simulink library "pwrsys"  (R2018a)
settings: Solver=VariableStepAuto  StartTime=0.0  StopTime=10.0  RelTol=1e-3
values from neighbouring files (symbols this model uses):
  Ts = Ts_c    (= 1e-07)    [PlantStateEquations_abc_Script.m]
undefined symbols (not defined in the file or in its folder): D1, Delta, DiscIntNeverNeededParam, ESS, f_LPF_noise, fn, fsw, grid, gt1, Iap, Kp, PCC, Refmax, Refmin, sim, SIMU, Sn, tctrl, Ti, Ts_control, Ts_PWM, Uabp, Uanp, WT, X, zeta
libraries: $bdroot x71, powerlib x59, powerlib_meascontrol x49, peTransforms x20, PhD_Library x1, sps_avr x1
(part 4 of 4)

== system pwrsys/Voltage and Current Controllers/DualRegulator ==
  idqref : Inport
  vabc : Inport  Port=2
  iabc : Inport  Port=3
  wt : Inport  Port=4
  w_pu : Inport  Port=5
  Udc : Inport  Port=6
  1=enable_acb : Inport  Port=7
  1=no,2=Notch,3=DSC : Inport  Port=8
  pre_mult_PI_errors : Inport  Port=9
  force_int : Inport  Port=10
  force_val : Inport  Port=11
  Bus Creator : BusCreator  Inputs=4
  Constant1 : Constant  Value=0
  Constant10 : Constant
  Constant14 : Constant
  Constant18 : Constant  Value=[0 0]
  Constant6 : Constant
  Constant8 : Constant  Value=0
  Idq_Dec_Signs_Fdbk_Ref : $bdroot/Voltage and Current Controllers/Idq_Dec_Signs_Fdbk_Ref  Ts=Ts  fn=fgrid  Kp=PI_Kp  Ti=PI_Ti  L=PI_X  PI_max=PI_max  PI_min=PI_min  TrafoPhaseComp=0
  Idq_Dec_Signs_Fdbk_Ref_acb : $bdroot/Voltage and Current Controllers/Idq_Dec_Signs_Fdbk_Ref  Ts=Ts  fn=fgrid  Kp=PI_Kp  Ti=PI_Ti  L=PI_X  PI_max=PI_max  PI_min=PI_min  TrafoPhaseComp=0
  PWM_abc_negwt_acb : $bdroot/PWM/PWM_abc_negwt_acb  fsw=PWM_fsw  Ts=PWM_Ts  Uabp=PWM_Uabp  PWM_Ini_Phase=PWM_Ini
  Selector1 : Selector  InputPortWidth=3  IndexOptions=Index vector (dialog)  Indices=[1 3 2]  OutputSizes=1
  Selector7 : Selector  InputPortWidth=3  IndexOptions=Index vector (dialog)  Indices=[1 3 2]  OutputSizes=1
  Terminator{1..4,24} (5 alike) : Terminator
  abc_dq_bypassnotch1 : $bdroot/Transformations/abc_dq_bypassnotch  Ts=Ts  fn=2*fgrid  fcutoutv=fcutoutLPF  fcutouti=fcutoutLPF  zeta=zetanotch
  abc_dq_bypassnotch2 : $bdroot/Transformations/abc_dq_bypassnotch  Ts=Ts  fn=2*fgrid  fcutoutv=fcutoutLPF  fcutouti=fcutoutLPF  zeta=zetanotch
  idqref_gen_for_cnst_p : $bdroot/Voltage and Current Controllers/idqref_gen_for_cnst_p  Ts_control=Ts
  PWMpulses : Outport
  Uabcref : Outport  Port=2
  mvidq : Outport  Port=3
  mpi+ : Outport  Port=4
  mpi- : Outport  Port=5
  wires:
  Udc/1 -> PWM_abc_negwt_acb/7
  abc_dq_bypassnotch1/1 -> idqref_gen_for_cnst_p/2, Bus Creator/3, Idq_Dec_Signs_Fdbk_Ref_acb/2  "vdq-"
  [w_pu] -> Idq_Dec_Signs_Fdbk_Ref/4
  PWM_abc_negwt_acb/3 -> Terminator24/1
  Constant14/1 -> Idq_Dec_Signs_Fdbk_Ref_acb/5
  abc_dq_bypassnotch2/1 -> idqref_gen_for_cnst_p/1, Bus Creator/1, Idq_Dec_Signs_Fdbk_Ref/2  "vdq+"
  abc_dq_bypassnotch1/2 -> Bus Creator/4, Idq_Dec_Signs_Fdbk_Ref_acb/3  "idq-"
  Constant10/1 -> PWM_abc_negwt_acb/2
  Constant8/1 -> PWM_abc_negwt_acb/4
  abc_dq_bypassnotch2/2 -> Bus Creator/2, Idq_Dec_Signs_Fdbk_Ref/3  "idq+"
  1=enable_acb/1 -> PWM_abc_negwt_acb/6
  Idq_Dec_Signs_Fdbk_Ref/1 -> PWM_abc_negwt_acb/1
  PWM_abc_negwt_acb/1 -> PWMpulses/1
  PWM_abc_negwt_acb/2 -> Uabcref/1  "Uabcref"
  Constant6/1 -> Idq_Dec_Signs_Fdbk_Ref/5
  Constant1/1 -> Idq_Dec_Signs_Fdbk_Ref_acb/6, Idq_Dec_Signs_Fdbk_Ref/6
  vabc/1 -> abc_dq_bypassnotch2/1, Selector7/1
  iabc/1 -> abc_dq_bypassnotch2/2, Selector1/1
  Idq_Dec_Signs_Fdbk_Ref_acb/1 -> PWM_abc_negwt_acb/5
  wt/1 -> abc_dq_bypassnotch2/3, abc_dq_bypassnotch1/3, [theta]
  Selector7/1 -> abc_dq_bypassnotch1/1
  Selector1/1 -> abc_dq_bypassnotch1/2
  Constant18/1 -> PWM_abc_negwt_acb/3
  idqref/1 -> idqref_gen_for_cnst_p/3, Idq_Dec_Signs_Fdbk_Ref/1
  idqref_gen_for_cnst_p/1 -> Idq_Dec_Signs_Fdbk_Ref_acb/1
  [theta] -> PWM_abc_negwt_acb/8
  1=no,2=Notch,3=DSC/1 -> abc_dq_bypassnotch2/5, abc_dq_bypassnotch1/5
  Bus Creator/1 -> mvidq/1
  w_pu/1 -> abc_dq_bypassnotch2/4, abc_dq_bypassnotch1/4, [w_pu]
  [w_pu] -> Idq_Dec_Signs_Fdbk_Ref_acb/4
  pre_mult_PI_errors/1 -> Idq_Dec_Signs_Fdbk_Ref_acb/7, Idq_Dec_Signs_Fdbk_Ref/7
  force_int/1 -> Idq_Dec_Signs_Fdbk_Ref_acb/8, Idq_Dec_Signs_Fdbk_Ref/8
  force_val/1 -> Idq_Dec_Signs_Fdbk_Ref_acb/10, Idq_Dec_Signs_Fdbk_Ref_acb/9, Idq_Dec_Signs_Fdbk_Ref/10, Idq_Dec_Signs_Fdbk_Ref/9
  Idq_Dec_Signs_Fdbk_Ref/4 -> mpi+/1
  Idq_Dec_Signs_Fdbk_Ref_acb/4 -> mpi-/1
  Idq_Dec_Signs_Fdbk_Ref/2 -> Terminator1/1
  Idq_Dec_Signs_Fdbk_Ref/3 -> Terminator2/1
  Idq_Dec_Signs_Fdbk_Ref_acb/2 -> Terminator3/1
  Idq_Dec_Signs_Fdbk_Ref_acb/3 -> Terminator4/1

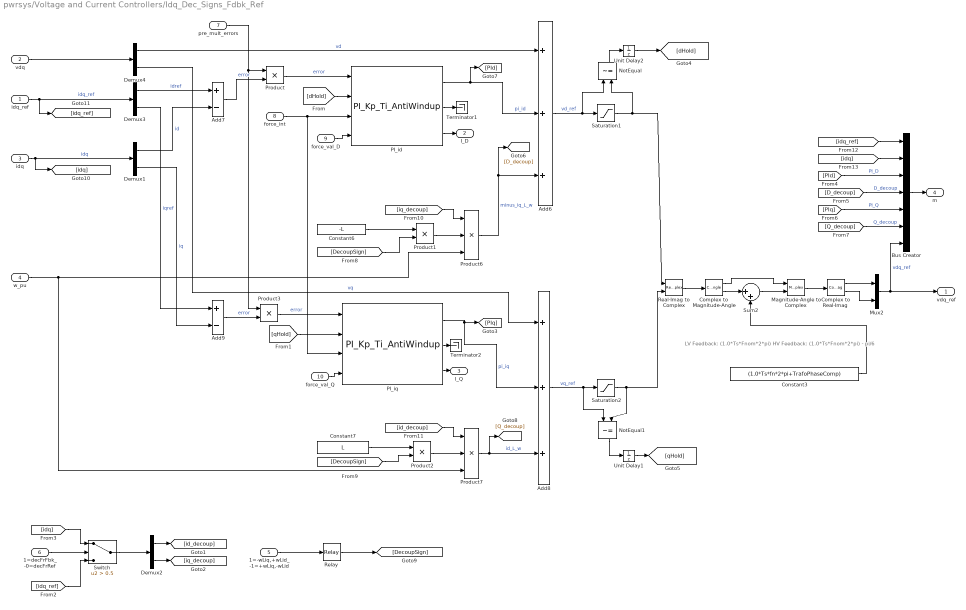
== system pwrsys/Voltage and Current Controllers/Idq_Dec_Signs_Fdbk_Ref ==
  note: LV Feedback: (1.0*Ts*Fnom*2*pi)
      | HV Feedback: (1.0*Ts*Fnom*2*pi) - pi/6
  idq_ref : Inport
  vdq : Inport  Port=2
  idq : Inport  Port=3
  w_pu : Inport  Port=4
  1=-wLiq,+wLid_-1=+wLiq,-wLid : Inport  Port=5
  1=decFrFbk_-0=decFrRef : Inport  Port=6
  pre_mult_errors : Inport  Port=7
  force_int : Inport  Port=8
  force_val_D : Inport  Port=9
  force_val_Q : Inport  Port=10
  Add6 : Sum  Inputs=+++
  Add7 : Sum  Inputs=+-
  Add8 : Sum  Inputs=+++
  Add9 : Sum  Inputs=+-
  Bus Creator : BusCreator  Inputs=7
  Complex to Magnitude-Angle : ComplexToMagnitudeAngle
  Complex to Real-Imag : ComplexToRealImag
  Constant3 : Constant  Value=(1.0*Ts*fn*2*pi+TrafoPhaseComp)  SampleTime=Ts
  Constant6 : Constant  Value=-L  SampleTime=Ts
  Constant7 : Constant  Value=L  SampleTime=Ts
  Demux{1..4} (4 alike) : Demux  Outputs=2
  Magnitude-Angle to Complex : MagnitudeAngleToComplex
  Mux2 : Mux  Inputs=2
  NotEqual : RelationalOperator  Operator=~=  OutDataTypeStr=boolean  RndMeth=Simplest
  NotEqual1 : RelationalOperator  Operator=~=  OutDataTypeStr=boolean  RndMeth=Simplest
  PI_id : $bdroot/Basic Blocks/PI_Kp_Ti_AntiWindup  Ts=Ts  Kp=Kp  Ti=Ti  PI_max=PI_max  PI_min=PI_min
  PI_iq : $bdroot/Basic Blocks/PI_Kp_Ti_AntiWindup  Ts=Ts  Kp=Kp  Ti=Ti  PI_max=PI_max  PI_min=PI_min
  Product : Product
  Product1 : Product  RndMeth=Zero
  Product2 : Product  RndMeth=Zero
  Product3 : Product
  Product6 : Product  Inputs=3  RndMeth=Zero
  Product7 : Product  Inputs=3  RndMeth=Zero
  Real-Imag to Complex : RealImagToComplex
  Relay : Relay  OnSwitchValue=0  OffSwitchValue=-0.1  OffOutputValue=-1
  Saturation1 : Saturate  UpperLimit=PI_max  LowerLimit=PI_min
  Saturation2 : Saturate  UpperLimit=PI_max  LowerLimit=PI_min
  Sum2 : Sum  Inputs=|++
  Switch : Switch  Criteria=u2 > Threshold  Threshold=0.5
  Terminator1 : Terminator
  Terminator2 : Terminator
  Unit Delay1 : UnitDelay  SampleTime=Ts
  Unit Delay2 : UnitDelay  SampleTime=Ts
  vdq_ref : Outport
  I_D : Outport  Port=2
  I_Q : Outport  Port=3
  m : Outport  Port=4
  wires:
  PI_iq/1 -> Add8/2, [PIq]  "pi_iq"
  PI_iq/2 -> Terminator2/1
  PI_id/2 -> Terminator1/1
  w_pu/1 -> Product7/3, Product6/3
  Product3/1 -> PI_iq/1  "error"
  PI_id/1 -> Add6/2, [PId]  "pi_id"
  Constant6/1 -> Product1/1
  Constant7/1 -> Product2/1
  Demux1/1 -> Add7/2  "id"
  Product7/1 -> [Q_decoup], Add8/3  "id_L_w"
  Demux4/1 -> Add6/1  "vd"
  Product/1 -> PI_id/1  "error"
  Demux1/2 -> Add9/2  "iq"
  Product6/1 -> [D_decoup], Add6/3  "minus_iq_L_w"
  PI_iq/3 -> I_Q/1
  PI_id/3 -> I_D/1
  Demux4/2 -> Add8/1  "vq"
  Mux2/1 -> Bus Creator/7, vdq_ref/1  "vdq_ref"
  idq/1 -> [idq], Demux1/1  "idq"
  vdq/1 -> Demux4/1
  Add8/1 -> NotEqual1/1, Saturation2/1  "vq_ref"
  Add6/1 -> NotEqual/1, Saturation1/1  "vd_ref"
  idq_ref/1 -> [idq_ref], Demux3/1  "idq_ref"
  Demux3/1 -> Add7/1  "idref"
  Demux3/2 -> Add9/1  "iqref"
  Magnitude-Angle to Complex/1 -> Complex to Real-Imag/1
  Real-Imag to Complex/1 -> Complex to Magnitude-Angle/1
  Complex to Magnitude-Angle/1 -> Magnitude-Angle to Complex/1
  Complex to Magnitude-Angle/2 -> Sum2/1
  Sum2/1 -> Magnitude-Angle to Complex/2
  Constant3/1 -> Sum2/2
  Complex to Real-Imag/1 -> Mux2/1
  Complex to Real-Imag/2 -> Mux2/2
  [PId] -> Bus Creator/3  "PI_D"
  [D_decoup] -> Bus Creator/4  "D_decoup"
  [PIq] -> Bus Creator/5  "PI_Q"
  Bus Creator/1 -> m/1
  [Q_decoup] -> Bus Creator/6  "Q_decoup"
  Saturation1/1 -> NotEqual/2, Real-Imag to Complex/1
  NotEqual/1 -> Unit Delay2/1
  Saturation2/1 -> NotEqual1/2, Real-Imag to Complex/2
  NotEqual1/1 -> Unit Delay1/1
  Unit Delay2/1 -> [dHold]
  Unit Delay1/1 -> [qHold]
  [dHold] -> PI_id/2
  [qHold] -> PI_iq/2
  Relay/1 -> [DecoupSign]
  1=-wLiq,+wLid_-1=+wLiq,-wLid/1 -> Relay/1
  [DecoupSign] -> Product1/2
  Product1/1 -> Product6/2
  Product2/1 -> Product7/2
  [DecoupSign] -> Product2/2
  [idq_ref] -> Switch/3
  Demux2/2 -> [iq_decoup]
  1=decFrFbk_-0=decFrRef/1 -> Switch/2
  Demux2/1 -> [id_decoup]
  Switch/1 -> Demux2/1
  [idq] -> Switch/1
  [iq_decoup] -> Product6/1
  [id_decoup] -> Product7/1
  [idq_ref] -> Bus Creator/1
  [idq] -> Bus Creator/2
  force_int/1 -> PI_iq/3, PI_id/3
  force_val_D/1 -> PI_id/4
  force_val_Q/1 -> PI_iq/4
  Add9/1 -> Product3/2  "error"
  Add7/1 -> Product/2  "error"
  pre_mult_errors/1 -> Product3/1, Product/1

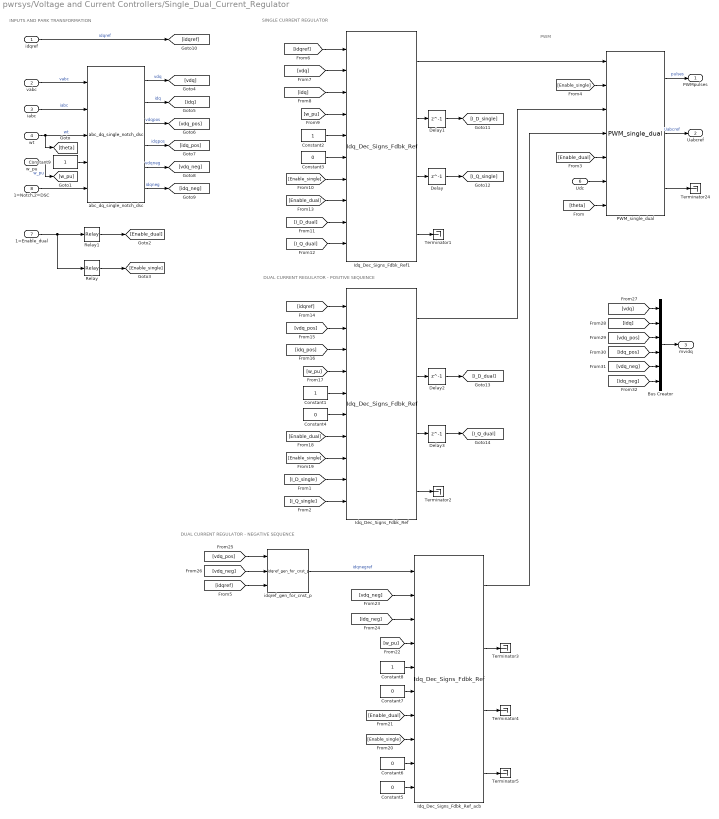
== system pwrsys/Voltage and Current Controllers/Single_Dual_Current_Regulator ==
  note: PWM
  note: DUAL CURRENT REGULATOR - NEGATIVE SEQUENCE
  note: DUAL CURRENT REGULATOR - POSITIVE SEQUENCE
  note: SINGLE CURRENT REGULATOR
  note: INPUTS AND PARK TRANSFORMATION
  idqref : Inport
  vabc : Inport  Port=2
  iabc : Inport  Port=3
  wt : Inport  Port=4
  w_pu : Inport  Port=5
  Udc : Inport  Port=6
  1=Enable_dual : Inport  Port=7
  1=Notch,2=DSC : Inport  Port=8
  Bus Creator : BusCreator  Inputs=6
  Constant{1..2,8..9} (4 alike) : Constant
  Constant{3..7} (5 alike) : Constant  Value=0
  Delay{,1..3} (4 alike) : Delay  DelayLength=1  InitialCondition=0  SampleTime=Ts
  Idq_Dec_Signs_Fdbk_Ref : $bdroot/Voltage and Current Controllers/Idq_Dec_Signs_Fdbk_Ref  Ts=Ts  fn=fgrid  Kp=PI_Kp  Ti=PI_Ti  L=PI_X  PI_max=PI_max  PI_min=PI_min  TrafoPhaseComp=0
  Idq_Dec_Signs_Fdbk_Ref1 : $bdroot/Voltage and Current Controllers/Idq_Dec_Signs_Fdbk_Ref  Ts=Ts  fn=fgrid  Kp=PI_Kp  Ti=PI_Ti  L=PI_X  PI_max=PI_max  PI_min=PI_min  TrafoPhaseComp=0
  Idq_Dec_Signs_Fdbk_Ref_acb : $bdroot/Voltage and Current Controllers/Idq_Dec_Signs_Fdbk_Ref  Ts=Ts  fn=fgrid  Kp=PI_Kp  Ti=PI_Ti  L=PI_X  PI_max=PI_max  PI_min=PI_min  TrafoPhaseComp=0
  PWM_single_dual : $bdroot/PWM/PWM_single_dual  fsw=PWM_fsw  Ts=PWM_Ts  Uabp=PWM_Uabp  PWM_Ini_Phase=PWM_Ini
  Relay : Relay  OnSwitchValue=0.6  OffSwitchValue=0.4  OnOutputValue=0  OffOutputValue=1
  Relay1 : Relay  OnSwitchValue=0.6  OffSwitchValue=0.4
  Terminator{1..5,24} (6 alike) : Terminator
  abc_dq_single_notch_dsc : $bdroot/Transformations/abc_dq_single_notch_dsc  Ts=Ts  fn=2*fgrid  zeta=zetanotch
  idqref_gen_for_cnst_p : $bdroot/Voltage and Current Controllers/idqref_gen_for_cnst_p  Ts_control=Ts
  PWMpulses : Outport
  Uabcref : Outport  Port=2
  mvidq : Outport  Port=3
  wires:
  Udc/1 -> PWM_single_dual/6
  PWM_single_dual/3 -> Terminator24/1
  PWM_single_dual/2 -> Uabcref/1  "Uabcref"
  [idqref] -> idqref_gen_for_cnst_p/3
  [theta] -> PWM_single_dual/7
  PWM_single_dual/1 -> PWMpulses/1  "pulses"
  1=Enable_dual/1 -> Relay1/1, Relay/1
  [Enable_dual] -> PWM_single_dual/5
  Relay/1 -> [Enable_single]
  [Enable_single] -> PWM_single_dual/2
  vabc/1 -> abc_dq_single_notch_dsc/1  "vabc"
  iabc/1 -> abc_dq_single_notch_dsc/2  "iabc"
  wt/1 -> [theta], abc_dq_single_notch_dsc/3  "wt"
  w_pu/1 -> [w_pu]  "w_pu"
  abc_dq_single_notch_dsc/1 -> [vdq]  "vdq"
  abc_dq_single_notch_dsc/2 -> [idq]  "idq"
  abc_dq_single_notch_dsc/3 -> [vdq_pos]  "vdqpos"
  abc_dq_single_notch_dsc/4 -> [idq_pos]  "idqpos"
  abc_dq_single_notch_dsc/5 -> [vdq_neg]  "vdqneg"
  abc_dq_single_notch_dsc/6 -> [idq_neg]  "idqneg"
  idqref/1 -> [idqref]  "idqref"
  [idqref] -> Idq_Dec_Signs_Fdbk_Ref1/1
  [vdq] -> Idq_Dec_Signs_Fdbk_Ref1/2
  [idq] -> Idq_Dec_Signs_Fdbk_Ref1/3
  [w_pu] -> Idq_Dec_Signs_Fdbk_Ref1/4
  Constant2/1 -> Idq_Dec_Signs_Fdbk_Ref1/5
  Constant3/1 -> Idq_Dec_Signs_Fdbk_Ref1/6
  Relay1/1 -> [Enable_dual]
  1=Notch,2=DSC/1 -> abc_dq_single_notch_dsc/5
  [Enable_single] -> Idq_Dec_Signs_Fdbk_Ref1/7
  Idq_Dec_Signs_Fdbk_Ref1/3 -> Delay/1
  Idq_Dec_Signs_Fdbk_Ref1/2 -> Delay1/1
  Idq_Dec_Signs_Fdbk_Ref/2 -> Delay2/1
  Idq_Dec_Signs_Fdbk_Ref/3 -> Delay3/1
  Delay1/1 -> [I_D_single]
  Delay/1 -> [I_Q_single]
  Delay2/1 -> [I_D_dual]
  Delay3/1 -> [I_Q_dual]
  [I_D_single] -> Idq_Dec_Signs_Fdbk_Ref/9
  [I_Q_single] -> Idq_Dec_Signs_Fdbk_Ref/10
  [I_D_dual] -> Idq_Dec_Signs_Fdbk_Ref1/9
  [I_Q_dual] -> Idq_Dec_Signs_Fdbk_Ref1/10
  [Enable_dual] -> Idq_Dec_Signs_Fdbk_Ref1/8
  [idqref] -> Idq_Dec_Signs_Fdbk_Ref/1
  [vdq_pos] -> Idq_Dec_Signs_Fdbk_Ref/2
  [idq_pos] -> Idq_Dec_Signs_Fdbk_Ref/3
  [w_pu] -> Idq_Dec_Signs_Fdbk_Ref/4
  Constant1/1 -> Idq_Dec_Signs_Fdbk_Ref/5
  Constant4/1 -> Idq_Dec_Signs_Fdbk_Ref/6
  [Enable_dual] -> Idq_Dec_Signs_Fdbk_Ref/7
  [Enable_single] -> Idq_Dec_Signs_Fdbk_Ref/8
  Idq_Dec_Signs_Fdbk_Ref1/4 -> Terminator1/1
  Idq_Dec_Signs_Fdbk_Ref/4 -> Terminator2/1
  Idq_Dec_Signs_Fdbk_Ref_acb/2 -> Terminator3/1
  Idq_Dec_Signs_Fdbk_Ref_acb/3 -> Terminator4/1
  Idq_Dec_Signs_Fdbk_Ref_acb/4 -> Terminator5/1
  Constant5/1 -> Idq_Dec_Signs_Fdbk_Ref_acb/10
  Constant6/1 -> Idq_Dec_Signs_Fdbk_Ref_acb/9
  [Enable_single] -> Idq_Dec_Signs_Fdbk_Ref_acb/8
  [Enable_dual] -> Idq_Dec_Signs_Fdbk_Ref_acb/7
  Constant7/1 -> Idq_Dec_Signs_Fdbk_Ref_acb/6
  Constant8/1 -> Idq_Dec_Signs_Fdbk_Ref_acb/5
  [w_pu] -> Idq_Dec_Signs_Fdbk_Ref_acb/4
  [vdq_neg] -> Idq_Dec_Signs_Fdbk_Ref_acb/2
  [idq_neg] -> Idq_Dec_Signs_Fdbk_Ref_acb/3
  [vdq_pos] -> idqref_gen_for_cnst_p/1
  [vdq_neg] -> idqref_gen_for_cnst_p/2
  idqref_gen_for_cnst_p/1 -> Idq_Dec_Signs_Fdbk_Ref_acb/1  "idqnegref"
  Idq_Dec_Signs_Fdbk_Ref1/1 -> PWM_single_dual/1
  Idq_Dec_Signs_Fdbk_Ref/1 -> PWM_single_dual/3
  Idq_Dec_Signs_Fdbk_Ref_acb/1 -> PWM_single_dual/4
  Bus Creator/1 -> mvidq/1
  [vdq] -> Bus Creator/1
  [idq] -> Bus Creator/2
  [vdq_pos] -> Bus Creator/3
  [idq_pos] -> Bus Creator/4
  [vdq_neg] -> Bus Creator/5
  [idq_neg] -> Bus Creator/6
  Constant9/1 -> abc_dq_single_notch_dsc/4

== system pwrsys/Voltage and Current Controllers/Uac_Controller ==
  vac_setpoint : Inport
  vac : Inport  Port=2
  Ihold : Inport  Port=3
  DisableP : Inport  Port=4
  pre_mult_error : Inport  Port=5
  force_int : Inport  Port=6
  force_val : Inport  Port=7
  PI_Kg_Kp_Ti_AntiWindup : $bdroot/Basic Blocks/PI_Kg_Kp_Ti_AntiWindup  Ts=Ts  Kg=Kg  Kp=Kp  Ti=Ti  PI_max=PI_max  PI_min=PI_min
  Product : Product
  Rate Transition1 : RateTransition  InitialCondition=1  OutPortSampleTime=Ts
  Rate Transition2 : RateTransition  InitialCondition=1  OutPortSampleTime=Ts
  Rate Transition3 : RateTransition  OutPortSampleTime=Ts
  Subtract : Sum  Inputs=+-
  Terminator2 : Terminator
  Terminator3 : Terminator
  iqref : Outport
  wires:
  PI_Kg_Kp_Ti_AntiWindup/2 -> Terminator2/1
  vac/1 -> Rate Transition1/1  "vac"
  PI_Kg_Kp_Ti_AntiWindup/3 -> Terminator3/1
  Subtract/1 -> Product/2
  Rate Transition1/1 -> Subtract/1
  Rate Transition2/1 -> Subtract/2
  PI_Kg_Kp_Ti_AntiWindup/1 -> iqref/1  "Idref"
  Ihold/1 -> PI_Kg_Kp_Ti_AntiWindup/3
  vac_setpoint/1 -> Rate Transition2/1
  DisableP/1 -> PI_Kg_Kp_Ti_AntiWindup/2
  force_val/1 -> PI_Kg_Kp_Ti_AntiWindup/5
  force_int/1 -> PI_Kg_Kp_Ti_AntiWindup/4
  pre_mult_error/1 -> Rate Transition3/1
  Rate Transition3/1 -> Product/1
  Product/1 -> PI_Kg_Kp_Ti_AntiWindup/1

== system pwrsys/Voltage and Current Controllers/Udc_Controller ==
  vdc : Inport
  Ihold : Inport  Port=2
  pre_mult_error : Inport  Port=3
  force_int : Inport  Port=4
  force_val : Inport  Port=5
  Constant1 : Constant
  PI_Kp_Ti_AntiWindup : $bdroot/Basic Blocks/PI_Kp_Ti_AntiWindup  Ts=Ts  Kp=Kp  Ti=Ti  PI_max=PI_max  PI_min=PI_min
  Product : Product
  Rate Transition1 : RateTransition  InitialCondition=1  OutPortSampleTime=Ts
  Rate Transition3 : RateTransition  OutPortSampleTime=Ts
  Subtract : Sum  Inputs=+-
  Terminator2 : Terminator
  Terminator3 : Terminator
  idref : Outport
  wires:
  PI_Kp_Ti_AntiWindup/2 -> Terminator2/1
  vdc/1 -> Rate Transition1/1  "vdc"
  PI_Kp_Ti_AntiWindup/3 -> Terminator3/1
  Subtract/1 -> Product/2
  Rate Transition1/1 -> Subtract/1
  Constant1/1 -> Subtract/2
  PI_Kp_Ti_AntiWindup/1 -> idref/1  "Idref"
  Ihold/1 -> PI_Kp_Ti_AntiWindup/2
  Rate Transition3/1 -> Product/1
  pre_mult_error/1 -> Rate Transition3/1
  Product/1 -> PI_Kp_Ti_AntiWindup/1
  force_int/1 -> PI_Kp_Ti_AntiWindup/3
  force_val/1 -> PI_Kp_Ti_AntiWindup/4

== system pwrsys/Voltage and Current Controllers/idqref_gen_for_cnst_p ==
  vdq+ : Inport
  vdq- : Inport  Port=2
  idqref : Inport  Port=3
  MATLAB Function : MATLAB Function  TreatAsAtomicUnit=on  SystemSampleTime=Ts
  idqref- : Outport
  wires:
  MATLAB Function/1(idqref) -> idqref-/1
  vdq+/1 -> MATLAB Function/1(vdqp)
  vdq-/1 -> MATLAB Function/2(vdqn)
  idqref/1 -> MATLAB Function/3("idqref ")

== system pwrsys/Voltage Sources/LSC_LCL_Trafo/INV_DClink ==
  CM : powerlib/Measurements/Current Measurement  PhasorSimulation=off  OutputType=Complex  PSBequivalent=0
  VM1 : powerlib/Measurements/Voltage Measurement  PhasorSimulation=off  OutputType=Complex  PSBequivalent=0
  Pin : PMIOPort  Side=Left
  Min : PMIOPort  Port=2  Side=Left
  Pout : PMIOPort  Port=3  Side=Right
  Mout : PMIOPort  Port=4  Side=Right
  Vdc : Outport
  Idc : Outport  Port=2
  wires:
  CM/1 -> Idc/1
  VM1/1 -> Vdc/1
  connections:
  VM1/LConn2 -- Mout/RConn1 -- Min/RConn1
  VM1/LConn1 -- CM/LConn1 -- Pin/RConn1
  CM/RConn1 -- Pout/RConn1

== system pwrsys/Voltage Sources/LSC_LCL_Trafo_AvgxSwitch/INV_DClink ==
  CM : powerlib/Measurements/Current Measurement  PhasorSimulation=off  OutputType=Complex  PSBequivalent=0
  VM1 : powerlib/Measurements/Voltage Measurement  PhasorSimulation=off  OutputType=Complex  PSBequivalent=0
  Pin : PMIOPort  Side=Left
  Min : PMIOPort  Port=2  Side=Left
  Pout : PMIOPort  Port=3  Side=Right
  Mout : PMIOPort  Port=4  Side=Right
  Vdc : Outport
  Idc : Outport  Port=2
  wires:
  CM/1 -> Idc/1
  VM1/1 -> Vdc/1
  connections:
  VM1/LConn2 -- Mout/RConn1 -- Min/RConn1
  VM1/LConn1 -- CM/LConn1 -- Pin/RConn1
  CM/RConn1 -- Pout/RConn1

== system pwrsys/Voltage Sources/SM_TG_EXC/Controllers ==
  deltaw : Inport
  Psp : Inport  Port=2
  Vref : Inport  Port=3
  Vm : Inport  Port=4
  Ifd : Inport  Port=5
  PSS : Inport  Port=6
  Active power x frequency droop GT1 : $bdroot/Basic Blocks/Droop controller  Refmax=SMcosphi  Refmin=0  Ts=1/(20*PCC.Fn)  Kp=GovKp  Kd=GovKd  Tr=GovTr  flp=GovFlp  DB=GovDB
  GT1 Excitation : sps_avr/ST1A Excitation System  Tr=ExcTr  KaTa=[ExcKa 1/(6*SMfn)]  VIminmax=[-0.2 0.2]  VAminmax=[ExcVRMin ExcVRMax]  VRminmax=[ExcVRMin ExcVRMax]  KfTf=[ExcKf ExcTf]  TbTc=[ExcTb ExcTc ExcTb1 ExcTc1]  KLR=0  ILR=999  Kc=0  v0=[1,(2/3)^0.5*1.57232]  TsBlock=1/(20*PCC.Fn)
      settings: SourceProductName=Simscape Power Systems  SourceProductBaseCode=PS
  GT1 P Comp pu : Constant  SampleTime=-1
  Rate Transition1 : RateTransition  OutPortSampleTime=1/(20*PCC.Fn)
  Rate Transition2 : RateTransition  OutPortSampleTime=1/(20*PCC.Fn)
  Rate Transition{3..6} (4 alike) : RateTransition
  Sum1 : Sum  Inputs=-+
  Turbine delay : DiscreteIntegrator  gainval=1/TurbT  InitialCondition=gt1.P.Ref  SampleTime=-1  LimitOutput=on  UpperSaturationLimit=SMcosphi  LowerSaturationLimit=0  ICPrevOutput=DiscIntNeverNeededParam  ICPrevScaledInput=DiscIntNeverNeededParam
  Pm : Outport
  Efd : Outport  Port=2
  wires:
  Vref/1 -> Rate Transition3/1
  Vm/1 -> Rate Transition4/1
  Active power x frequency droop GT1/1 -> Sum1/2  "PrefGT1"
  Rate Transition6/1 -> GT1 Excitation/4
  Turbine delay/1 -> Pm/1, Sum1/1  "Pm"
  GT1 Excitation/1 -> Efd/1  "Efd"
  GT1 P Comp pu/1 -> Active power x frequency droop GT1/3
  Ifd/1 -> Rate Transition5/1
  Sum1/1 -> Turbine delay/1
  Psp/1 -> Rate Transition1/1
  deltaw/1 -> Rate Transition2/1
  Rate Transition2/1 -> Active power x frequency droop GT1/1
  Rate Transition1/1 -> Active power x frequency droop GT1/2
  Rate Transition3/1 -> GT1 Excitation/1
  Rate Transition4/1 -> GT1 Excitation/2
  Rate Transition5/1 -> GT1 Excitation/3
  PSS/1 -> Rate Transition6/1

== matlab function pwrsys/Adaptive Moving Averages/AMA with insertion pointer driven buffer/MATLAB Function ==
  data: x input; xavg output; n input; Nb input; xacc output; xdec output
%%%%%%%%%%%%%%%%%%%%%%%%%%%%%%%%%%%%%%%%%%%%%%%%%%%%%%%%%%%%%%%%%%%%%%%%%%
% Adaptive Moving Average Block
%%%%%%%%%%%%%%%%%%%%%%%%%%%%%%%%%%%%%%%%%%%%%%%%%%%%%%%%%%%%%%%%%%%%%%%%%%
function [xavg, xacc, xdec]  = AMAInsertionPntrDriven( x, n, Nb)

persistent buffer bufferlen rzero izero rone ione Nb_fix xavg_internal nold
 
for_acc_internal = 0;
for_dec_internal = 0;

%%%%%%%%%%%%%%%%%%%%%%%%%%%%%%%%%%
% Values of at the first cycle
%%%%%%%%%%%%%%%%%%%%%%%%%%%%%%%%%%
if isempty(buffer)
    %Nb should be larger than 2
    if Nb < 1
        %lenght of the buffer is Nb+1
        Nb_fix = 1;
        bufferlen = 2;
    else
        Nb_fix = round(Nb); %lenght of the buffer is Nb+1
        bufferlen = Nb_fix + 1;
    end
    
    %create the buffer with zeros 
    buffer = zeros(bufferlen,1);
    
    %check is n smaller or equal to Nb
    if n > Nb_fix
        n = Nb_fix;
    else
        if n < 1
            n = 1; 
        else
            n = round(n);
        end
    end
    
    %initialize pointers
    rzero = 0;
    izero = rzero + n;
    
    rone = rzero + 1;
    ione = izero + 1;
    
    %first insertion 
    %bufferlen = Nb+1 so I can write to the buffer first
    buffer(ione) = x/n;
    
    %calculating value for accumulation
    for_acc_internal = x/n;
    for_dec_internal = 0;
    
    %accumulator
    xavg_internal = for_acc_internal; 
    nold = n;
else
%%%%%%%%%%%%%%%%%%%%%%%%%%%%%%%%%%
% Here the function starts actually
%%%%%%%%%%%%%%%%%%%%%%%%%%%%%%%%%%
    %check if n smaller or equal to Nb
    if n > Nb_fix
        n = Nb_fix;
    else
        if n < 1
            n = 1; 
        else
            n = round(n);
        end
    end
    
    %insertion pointer moves forward, slot is replaced
    %bufferlen = Nb+1 so I can write to the buffer first
    izero = round( mod(izero + 1, bufferlen));
    ione = izero + 1;
    buffer(ione) = x/n;
    for_acc_internal = x/n; 
    
    %retrieval logic
    if n >= nold
        %retrieval pointer can jump backwards (as I had zeroed the buffer
        %after retrievals)
        rzero = round( mod(izero - n, bufferlen));
        rone = rzero + 1;
        for_dec_internal = buffer(rone);
        buffer(rone) = 0;
        nold = n;
    else
        jump = nold - n;
        for aux=0:jump
            rzero = round( mod(rzero + 1, bufferlen));
            rone = rzero + 1;
            for_dec_internal = for_dec_internal + buffer(rone);
            buffer(rone) = 0;
            nold = n;
        end
    end
    
    %accumulation
    xavg_internal = xavg_internal + for_acc_internal - for_dec_internal; 
end

xacc = for_acc_internal;
xdec = for_dec_internal;
xavg = xavg_internal;

== matlab function pwrsys/Adaptive Moving Averages/AMA with retrieval pointer driven buffer/MATLAB Function ==
  data: x input; xavg output; n input; Nb input; xacc output; xdec output
%%%%%%%%%%%%%%%%%%%%%%%%%%%%%%%%%%%%%%%%%%%%%%%%%%%%%%%%%%%%%%%%%%%%%%%%%%
% Adaptive Moving Average Block
%%%%%%%%%%%%%%%%%%%%%%%%%%%%%%%%%%%%%%%%%%%%%%%%%%%%%%%%%%%%%%%%%%%%%%%%%%
% Prog/rev history
%   Mota - 2020-11-24: first release
function [xavg, xacc, xdec]  = AMARetrievalPntrDriven( x, n, Nb)

persistent buffer bufferlen r i Nb_fix xavg_internal

for_acc_internal = 0;
for_dec_internal = 0;

%%%%%%%%%%%%%%%%%%%%%%%%%%%%%%%%%%
% Values at the first cycle
%%%%%%%%%%%%%%%%%%%%%%%%%%%%%%%%%%
if isempty(buffer)
    %Nb should be larger than 1
    if Nb < 1
        %lenght of the buffer is Nb+1
        Nb_fix = 1;
        bufferlen = 2;
    else
        Nb_fix = round(Nb); %lenght of the buffer is Nb+1
        bufferlen = Nb_fix + 1;
    end
    
    %create the buffer with zeros 
    buffer = zeros(bufferlen,1);
    
    %check is n smaller or equal to Nb
    if n > Nb_fix
        n = Nb_fix;
    else
        if n < 1
            n = 1; 
        else
            n = round(n);
        end
    end
    
    %initialize pointers
    r = 1;
    i = r + n;
    
    %first sum 
    buffer(i) = buffer(i) + x/n;
    
    %calculating value for accumulation
    for_acc_internal = x/n;
    for_dec_internal = 0;
    
    %accumulator
    %xavg_internal = for_acc_internal - for_dec_internal; %first cycle, for_dec_internal=0
    xavg_internal = for_acc_internal; 
else
%%%%%%%%%%%%%%%%%%%%%%%%%%%%%%%%%%
% Here the function starts actually
%%%%%%%%%%%%%%%%%%%%%%%%%%%%%%%%%%
    %check if n smaller or equal to Nb
    if n > Nb_fix
        n = Nb_fix;
    else
        if n < 1
            n = 1; 
        else
            n = round(n);
        end
    end
    
    %pointer update
    r = r + 1;
    r = round( mod(r - 1, bufferlen) + 1); %mod works with index starting at zero, but matlab works with index on 1 
    i = round( mod(r - 1 + n, bufferlen) + 1);
    
    %insertion (sum)
    for_acc_internal = x/n; 
    buffer(i) = buffer(i) + for_acc_internal;
        
    %retrieval and zeroing 
    for_dec_internal = buffer(r);
    buffer(r) = 0; 
    
    %accumulation
    xavg_internal = xavg_internal + for_acc_internal - for_dec_internal; 
end

xacc = for_acc_internal;
xdec = for_dec_internal;
xavg = xavg_internal;

== matlab function pwrsys/Adaptive Moving Averages/Subsystem/MATLAB Function ==
  data: x input; xavg output; xavground output; n input; Nb input; xavgceil output; xavgfloor output; xavgweigthed output; nr output; nf output; nc output; changecnt output
%%%%%%%%%%%%%%%%%%%%%%%%%%%%%%%%%%%%%%%%%%%%%%%%%%%%%%%%%%%%%%%%%%%%%%%%%%
% Adaptive Moving Average Block
%%%%%%%%%%%%%%%%%%%%%%%%%%%%%%%%%%%%%%%%%%%%%%%%%%%%%%%%%%%%%%%%%%%%%%%%%%
% Prog/rev history
%   Mota - 2020-12-08: first release

function [xavg, xavground, xavgceil, xavgfloor, xavgweigthed, nr, nf, nc, changecnt]  = AMARetrievalPntrDriven( x, n, Nb)

persistent bufferlen Nb_fix
persistent bufferround nround rround iround
persistent bufferceil nceil rceil iceil
persistent bufferfloor nfloor rfloor ifloor
persistent xavg_internal_ceil xavg_internal_round xavg_internal_floor
persistent old_nceil k_change_counter

for_acc_internal_ceil = 0;
for_dec_internal_ceil = 0;

for_acc_internal_round = 0;
for_dec_internal_round = 0;

for_acc_internal_floor = 0;
for_dec_internal_floor = 0;

nnow = n; 

%%%%%%%%%%%%%%%%%%%%%%%%%%%%%%%%%%
% Values of at the first cycle
%%%%%%%%%%%%%%%%%%%%%%%%%%%%%%%%%%
if isempty(bufferceil)
    %Nb should be larger than 1
    if Nb < 1
        %lenght of the buffer is Nb+1
        Nb_fix = 1;
        bufferlen = 2;
    else
        Nb_fix = round(Nb);%lenght of the buffer is Nb+1
        bufferlen = round(Nb_fix+1);
    end
    
    %initialize the buffer
    bufferceil = zeros(bufferlen,1);
    bufferround = zeros(bufferlen,1);
    bufferfloor = zeros(bufferlen,1);
    
    %check is n smaller or equal to Nb
    if nnow > Nb_fix
        nnow = Nb_fix;
        nceil = Nb_fix;
        nround = Nb_fix;
        nfloor = Nb_fix;
    else
        if nnow < 1
            nnow = 1;
            nceil = 1;
            nround = 1;
            nfloor = 1;
        else
            nceil = ceil(nnow);
            nround = round(nnow);
            nfloor = floor(nnow);
        end
    end
    
    %detecting change in ceiling
    old_nceil = nceil;
    k_change_counter = 0; 
    
    %initialize pointers
    rceil = 1;
    iceil = rceil + nceil;
    
    rround = 1;
    iround = rround + nround;
        
    rfloor = 1;
    ifloor = rfloor + nfloor;
        
    %first sum 
    bufferceil(iceil) = bufferceil(iceil) + x/nceil;
    bufferround(iround) = bufferround(iround) + x/nround;
    bufferfloor(ifloor) = bufferfloor(ifloor) + x/nfloor;
    
    %calculating value for accumulation
    for_acc_internal_ceil  = x/nceil;
    for_dec_internal_ceil = 0;
    
    for_acc_internal_round  = x/nround;
    for_dec_internal_round = 0;        
    
    for_acc_internal_floor  = x/nfloor;
    for_dec_internal_floor = 0;
        
    %accumulator
    xavg_internal_ceil = for_acc_internal_ceil; 
    xavg_internal_round = for_acc_internal_round; 
    xavg_internal_floor = for_acc_internal_floor; 
else
%%%%%%%%%%%%%%%%%%%%%%%%%%%%%%%%%%
% Here the function starts actually
%%%%%%%%%%%%%%%%%%%%%%%%%%%%%%%%%%
    %check is n smaller or equal to Nb
    if nnow > Nb_fix
        nnow = Nb_fix;
        nceil = Nb_fix;
        nround = Nb_fix;
        nfloor = Nb_fix;
    else
        if nnow < 1
            nnow = 1;
            nceil = 1;
            nround = 1;
            nfloor = 1;
        else
            nceil = ceil(nnow);
            nround = round(nnow);
            nfloor = floor(nnow);
        end
    end
    
    %pointer update
    %mod works from zero, matlab arrays start at index 1
    rceil = rceil + 1;
    rceil = round( mod(rceil - 1, bufferlen)+1); 
    iceil = round( mod(rceil - 1 + nceil, bufferlen) + 1);

    rround = rround + 1;
    rround = round( mod(rround - 1, bufferlen)+1); 
    iround = round( mod(rround - 1 + nround, bufferlen) + 1);
    
    rfloor = rfloor + 1;
    rfloor = round( mod(rfloor - 1, bufferlen)+1); 
    ifloor = round( mod(rfloor - 1 + nfloor, bufferlen) + 1);

    %insertion (sum)
    for_acc_internal_ceil = x/nceil; 
    bufferceil(iceil) = bufferceil(iceil) + for_acc_internal_ceil;

    for_acc_internal_round = x/nround; 
    bufferround(iround) = bufferround(iround) + for_acc_internal_round;
    
    for_acc_internal_floor = x/nfloor; 
    bufferfloor(ifloor) = bufferfloor(ifloor) + for_acc_internal_floor;

    
    %retrieval and zeroing 
    for_dec_internal_ceil = bufferceil(rceil);
    bufferceil(rceil) = 0; 

    for_dec_internal_round = bufferround(rround);
    bufferround(rround) = 0; 
        
    for_dec_internal_floor = bufferfloor(rfloor);
    bufferfloor(rfloor) = 0; 
    
    
    %accumulation
    xavg_internal_ceil = xavg_internal_ceil + for_acc_internal_ceil - for_dec_internal_ceil; 
    xavg_internal_round = xavg_internal_round + for_acc_internal_round - for_dec_internal_round; 
    xavg_internal_floor = xavg_internal_floor + for_acc_internal_floor - for_dec_internal_floor; 
end

xavgceil = xavg_internal_ceil;
xavground = xavg_internal_round;
xavgfloor = xavg_internal_floor;
xavgweigthed = (nnow - nfloor) * xavg_internal_ceil + (1 - nnow + nfloor) * xavg_internal_floor;
%alpha = (nnow - nfloor);
%oneminusalpha = (1 - nnow + nfloor);

nr = nround;
nf = nfloor;
nc = nceil;
changenc = 0;

%Check for changes in nceil and start a timer
if old_nceil ~= nceil
    changenc = 1;
    k_change_counter = 1; 
else
    if k_change_counter > 0
        k_change_counter = k_change_counter  + 1;
        if k_change_counter > nceil
            changenc = 0; 
            k_change_counter = 0;
        else
            changenc = 1;
        end
    end
end

if changenc == 1
    xavg = xavg_internal_round;
else
    xavg = (nnow - nfloor) * xavg_internal_ceil + (1 - nnow + nfloor) * xavg_internal_floor;
end
old_nceil = nceil;
changecnt = k_change_counter;

== matlab function pwrsys/Voltage and Current Controllers/idqref_gen_for_cnst_p/MATLAB Function ==
  data: vdqp input; idqref output; vdqn input; idqref input
function idqref = fcn(vdqp,vdqn,idqref)

% Calculation of the negative sequence references for zeroing the active 
% power second harmonic oscillations
% 
% Derived independently from, but later noticed that the same line of
% reasoning was adopted by Chaudhary 2012 "Negative Sequence Current
% Control in Wind Power Plants With VSC-HVDC Connection"

% In "expanded" matrix form
% | idn | = - | -vdp  +vqp |^{-1} * | -vdn  +vqn | * | idp | 
% | iqn | =   | +vqp  +vdp |        | -vdn  +vqn |   | idq |
% In matrix form
%  idqn   = -   vdqp^{-1}         *      vdqn      *   idqp

%The matrix that will be inverted
vp = zeros(2);
vp(1,1) = -vdqp(1);
vp(1,2) = vdqp(2);
vp(2,1) = vdqp(2);
vp(2,2) = vdqp(1);

%The matrix that is not inverted
vn = zeros(2);
vn(1,1) = -vdqn(1);
vn(1,2) = vdqn(2);
vn(2,1) = vdqn(2);
vn(2,2) = vdqn(1);

% idqn = - vdqp^{-1} * vdqn * idqp
idqref = -vp\vn*idqref;

== matlab function pwrsys/Basic Blocks/digital_integrator/MATLAB Function ==
  data: x input; y output; max input; min input; force input; forceval input; Ts input
%%%%%%%%%%%%%%%%%%%%%%%%%%%%%%%%%%%%%%%%%%%%%%%%%%%%%%%%%%%%%%%%%%%%%%%%%%
% Digital integrator
%%%%%%%%%%%%%%%%%%%%%%%%%%%%%%%%%%%%%%%%%%%%%%%%%%%%%%%%%%%%%%%%%%%%%%%%%%\
% Forward Euler method: as in matlab help
%   y(n) = y(n-1) + Ts(n-1)*x(n-1)
%   used it to avoid algebraic loops
%
% All inputs are stored in states, so there is no direct feedthrough
% Workaround to avoid algebraic loops
% see: https://www.mathworks.com/help/simulink/ug/integration-considerations-for-matlab-function-blocks.html
%
% Inputs
%   x: input to the integrator
%   max: max value for integrator
%   min: min value for integrator
%   force: if=1 sets integrator to forceval
%   forceval: see line above (max and min are respected
%   Ts: sampling time
% Output
%   y: output of the integrator
%
%%%%%%%%%%%%%%%%%%%%%%%%%%%%%%%%%%%%%%%%%%%%%%%%%%%%%%%%%%%%%%%%%%%%%%%%%%\
% Prog/rev history
%   Mota - 2021-05-21: first release

function y = DigInt(x, max, min, force, forceval, Ts)

% The value of the integrator
persistent i
persistent old_x
persistent old_max
persistent old_min
persistent old_force
persistent old_forceval
persistent old_Ts

% Only at first cycle - outputs zero
if isempty(i)
    y = 0;
    i = 0;
    old_x = 0;
    old_max = 0;
    old_min = 0;
    old_force = 0;
    old_forceval = 0;
    old_Ts = 0;
    % On the second cycle, output will still be zero, due to choices above
    return;
end

% auxiliary value
aux = 0;

% Bypassing the integrator with a value (can be used for followup)
if old_force == 1
    aux = old_forceval;
else
    %if not bypass, then calculate the next value of the integrator
    aux = i + old_Ts*old_x;
end

%Limiting the integrator
if aux > old_max
    % max value has priority, i.e.,
    % if "max" is below "min" due to engineer error
    % the integrator will stop at "max"
    aux = old_max;
elseif aux < old_min
    % if integrator would cross the min, it will be stopped at min
    aux = old_min;
end

% output of the integrator
y = aux;

%update states
i = aux;
old_x = x;
old_max = max;
old_min = min;
old_force = force;
old_forceval = forceval;
old_Ts = Ts;

== matlab function pwrsys/Basic Blocks/digital_ramp_gen/MATLAB Function ==
  data: up input; down input; rate input; y output; max input; min input; force input; forceval input; Ts input
%%%%%%%%%%%%%%%%%%%%%%%%%%%%%%%%%%%%%%%%%%%%%%%%%%%%%%%%%%%%%%%%%%%%%%%%%%
% Digital integrator
%%%%%%%%%%%%%%%%%%%%%%%%%%%%%%%%%%%%%%%%%%%%%%%%%%%%%%%%%%%%%%%%%%%%%%%%%%\
% Forward Euler method: as in matlab help
%   y(n) = y(n-1) + Ts(n-1)*x(n-1)
%   uset it to avoid algebraic loops

% All inputs are stored in states, so there is no direct feedthrough
% GAMBIARRA for avoiding algebraic loops
% see: https://www.mathworks.com/help/simulink/ug/integration-considerations-for-matlab-function-blocks.html

% Inputs
%   up: ramps up
%   down: ramps down (if both up and down, than stops)
%   max: max value for ramp
%   min: min value for ramp
%   force: if=1 sets integrator to forceval
%   forceval: see line above (max and min are respected
%   Ts: sampling time
% Output
%   y: output of the ramp

%%%%%%%%%%%%%%%%%%%%%%%%%%%%%%%%%%%%%%%%%%%%%%%%%%%%%%%%%%%%%%%%%%%%%%%%%%\
% Prog/rev history
%   Mota - 2021-05-21: first release

function y = DigRamp(up, down, rate, max, min, force, forceval, Ts)

% The value of the integrator
persistent i
persistent old_up
persistent old_down
persistent old_rate
persistent old_max
persistent old_min
persistent old_force
persistent old_forceval
persistent old_Ts

% Only at first cycle - outputs zero
if isempty(i)
    y = 0;
    i = 0;
    old_up = 0;
    old_down = 0;
    old_rate = 0;
    old_max = 0;
    old_min = 0;
    old_force = 0;
    old_forceval = 0;
    old_Ts = 0;
    % On the second cycle, output will still be zero, due to choices above
    return;
end

% auxiliary value
aux = 0;

% Bypassing the integrator with a value (can be used for followup)
if old_force == 1
    aux = old_forceval;
else
    %if not bypass, then calculate the next value of the integrator
    aux = i + old_Ts*old_rate*old_up + old_Ts*old_rate*old_down ;
end

%Limiting the integrator
if aux > old_max
    % max value has priority, i.e.,
    % if "max" is below "min" due to engineer error
    % the integrator will stop at "max"
    aux = old_max;
elseif aux < old_min
    % if integrator would cross the min, it will be stopped at min
    aux = old_min;
end

% output of the integrator
y = aux;

%update states
i = aux;
old_rate = rate;
%ramps up if up > 0
if up > 0
    old_up = 1;
else
    old_up = 0;
end
%ramps down if down > 0
if down > 0 
    old_down = -1;
else
    old_down = 0;
end
old_max = max;
old_min = min;
old_force = force;
old_forceval = forceval;
old_Ts = Ts;
